simulink model "nid_skeleton_eML"  (Simulink 10.0)
settings: Solver=FixedStepDiscrete  StartTime=0.0  StopTime=inf  RelTol=1e-3  EnableMultiTasking=on
libraries: nid_lib x2
settings Model: Creator=tchikama  LastModifiedBy=bhisma
settings DataIOCC: LimitDataPoints=on  SignalLoggingSaveFormat=ModelDataLogs  SaveOutput=off
settings OptimizationCC: ExpressionDepthLimit=2147483647  SimCompilerOptimization=on
settings DebuggingCC: SolverPrmCheckMsg=warning  FcnCallInpInsideContextMsg=warning  StateNameClashWarn=warning
settings HardwareCC: ProdIntDivRoundTo=Zero  ProdEndianess=LittleEndian  ProdHWDeviceType=Generic->32-bit x86 compatible
settings RTWCC: RTWCompilerOptimization=on
settings CodeAppCC: MaxIdLength=95
settings GRTTargetCC: GeneratePreprocessorConditionals=Disable all
settings ConfigComp: CovExternalEMLEnable=off

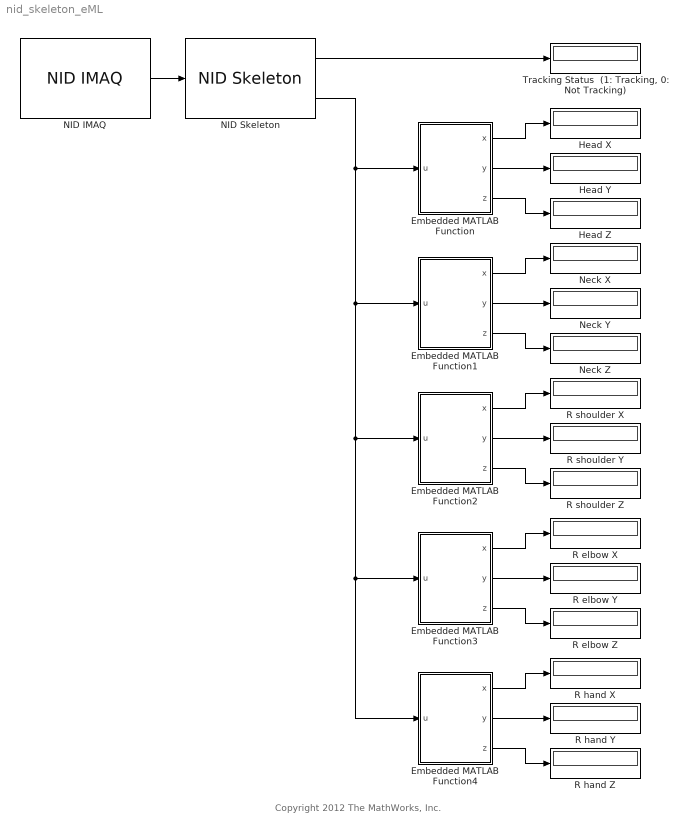
== system nid_skeleton_eML ==
  note: Copyright 2012 The MathWorks, Inc.
  Embedded MATLAB Function : MATLAB Function  TreatAsAtomicUnit=on
  Embedded MATLAB Function1 : MATLAB Function  TreatAsAtomicUnit=on
  Embedded MATLAB Function2 : MATLAB Function  TreatAsAtomicUnit=on
  Embedded MATLAB Function3 : MATLAB Function  TreatAsAtomicUnit=on
  Embedded MATLAB Function4 : MATLAB Function  TreatAsAtomicUnit=on
  Head X : Display
  Head Y : Display
  Head Z : Display
  NID IMAQ : nid_lib/NID IMAQ  imaq_depth=off  imaq_motion=off  imaq_image=off  view_point=off  imaq_skeleton=on  imaq_ir=off  mirror_image=off  imaq_sample_time=1/30  res_fps=VGA (640x480): 30 FPS  needPsiPose=off  angle=0  angle_read=off  near_mode=off
  NID Skeleton : nid_lib/NID Skeleton  num_of_skeleton_tracking=1  conv_XYZ_RW=on  viewer=off
  Neck X : Display
  Neck Y : Display
  Neck Z : Display
  R elbow X : Display
  R elbow Y : Display
  R elbow Z : Display
  R hand X : Display
  R hand Y : Display
  R hand Z : Display
  R shoulder X : Display
  R shoulder Y : Display
  R shoulder Z : Display
  "Tracking Status  (1: Tracking, 0: Not Tracking)" : Display
  wires:
  NID IMAQ/1 -> NID Skeleton/1
  NID Skeleton/2 -> Embedded MATLAB Function3/1(u), Embedded MATLAB Function4/1(u), Embedded MATLAB Function2/1(u), Embedded MATLAB Function1/1(u), Embedded MATLAB Function/1(u)
  NID Skeleton/1 -> "Tracking Status  (1: Tracking, 0: Not Tracking)"/1
  Embedded MATLAB Function/1(x) -> Head X/1
  Embedded MATLAB Function/2(y) -> Head Y/1
  Embedded MATLAB Function/3(z) -> Head Z/1
  Embedded MATLAB Function1/1(x) -> Neck X/1
  Embedded MATLAB Function1/2(y) -> Neck Y/1
  Embedded MATLAB Function1/3(z) -> Neck Z/1
  Embedded MATLAB Function2/1(x) -> R shoulder X/1
  Embedded MATLAB Function2/2(y) -> R shoulder Y/1
  Embedded MATLAB Function2/3(z) -> R shoulder Z/1
  Embedded MATLAB Function3/1(x) -> R elbow X/1
  Embedded MATLAB Function3/2(y) -> R elbow Y/1
  Embedded MATLAB Function3/3(z) -> R elbow Z/1
  Embedded MATLAB Function4/1(x) -> R hand X/1
  Embedded MATLAB Function4/2(y) -> R hand Y/1
  Embedded MATLAB Function4/3(z) -> R hand Z/1

== matlab function Embedded MATLAB Function1 ==
  data: x output double; u input double; y output double; z output double
function [x,y,z] = fcn(u)
%#eml

%
% Neck
%
if length(u) == 20
    idx = 3; % Kinect SDK
else
    idx = 2; % OpenNI
end

x = u(:,idx,1);
y = u(:,idx,2);
z = u(:,idx,3);

== matlab function Embedded MATLAB Function ==
  data: x output double; u input double; y output double; z output double
function [x,y,z] = fcn(u)
%#eml

%
% Head
%
if length(u) == 20
    idx = 4; % Kinect SDK
else
    idx = 1; % OpenNI
end

x = u(:,idx,1);
y = u(:,idx,2);
z = u(:,idx,3);

== matlab function Embedded MATLAB Function2 ==
  data: x output double; u input double; y output double; z output double
function [x,y,z] = fcn(u)
%#eml

%
% Right shoulder
%
if length(u) == 20
    idx = 9; % Kinect SDK
else
    idx = 4; % OpenNI
end

x = u(:,idx,1);
y = u(:,idx,2);
z = u(:,idx,3);

== matlab function Embedded MATLAB Function3 ==
  data: x output double; u input double; y output double; z output double
function [x,y,z] = fcn(u)
%#eml

%
% Right elbow
%
if length(u) == 20
    idx = 10; % Kinect SDK
else
    idx = 5; % OpenNI
end

x = u(:,idx,1);
y = u(:,idx,2);
z = u(:,idx,3);

== matlab function Embedded MATLAB Function4 ==
  data: x output double; u input double; y output double; z output double
function [x,y,z] = fcn(u)
%#eml

%
% Right hand
%
if length(u) == 20
    idx = 12; % Kinect SDK
else
    idx = 6; % OpenNI
end

x = u(:,idx,1);
y = u(:,idx,2);
z = u(:,idx,3);
